simulink model "Woche02_A2"  (R2016a)
settings: Solver=VariableStepAuto  StartTime=0.0  StopTime=100  RelTol=1e-3
values from neighbouring files (symbols this model uses):
  n = lambda*tEnd    [Woche02_A1.m]
undefined symbols (not defined in the file or in its folder): m
settings Model: Creator=gome  LastModifiedBy=gome

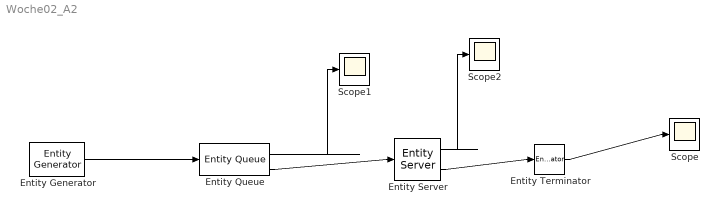
== system Woche02_A2 ==
  Entity Generator : EntityGenerator  OutputPortMessageModes=m  TimeSource=MATLAB action  IntergenerationTimeAction=dt = exprnd(0.1);  EntityType=Structured  EntityTypeName=Entity
  Entity Queue : EntityQueue  InputPortMessageModes=m  OutputPortMessageModes=n,m  Capacity=inf  NumberEntitiesInBlock=on
      settings: OutputPortMap=o1,o5
  Entity Server : EntityServer  InputPortMessageModes=m  OutputPortMessageModes=n,m  Capacity=1  ServiceTimeSource=MATLAB action  ServiceTimeAction=dt = 10/60*rand(1,1);  Utilization=on
      settings: OutputPortMap=o5,o9
  Entity Terminator : EntityTerminator  InputPortMessageModes=m  NumberEntitiesArrived=on
      settings: OutputPortMap=o0
  Scope : Scope
  Scope1 : Scope
  Scope2 : Scope
  wires:
  Entity Generator/1 -> Entity Queue/1
  Entity Terminator/1 -> Scope/1
  Entity Server/2 -> Entity Terminator/1
  Entity Queue/2 -> Entity Server/1
  Entity Queue/1 -> Scope1/1
  Entity Server/1 -> Scope2/1
